simulink model "poles5_rocky"  (R2022a)
settings: Solver=VariableStepAuto  StartTime=0.0  StopTime=5  RelTol=1e-3
values from neighbouring files (symbols this model uses):
  a = 10.12    [poles3_calculate.m]    (also in poles5_calculate.m; poles_calculate.m = 10.33)
  b = 0.00301    [poles3_calculate.m]    (also in poles5_calculate.m; poles_calculate.m = 0.0029)
  Ci_simulink = real(Ci)    [poles5_calculate.m]
  g = 9.81    [poles3_calculate.m]    (also in poles5_calculate.m; poles_calculate.m)
  Ji_simulink = real(Ji)    [poles5_calculate.m]
  Jp_simulink = real(Jp)    [poles5_calculate.m]
  Ki_simulink = real(Ki)    [poles5_calculate.m]
  Kp_simulink = real(Kp)    [poles5_calculate.m]
  l = 0.40038    [poles3_calculate.m]    (also in poles5_calculate.m; poles_calculate.m = 0.4168)
settings Model: Creator=cpark1  LastModifiedBy=cpark1

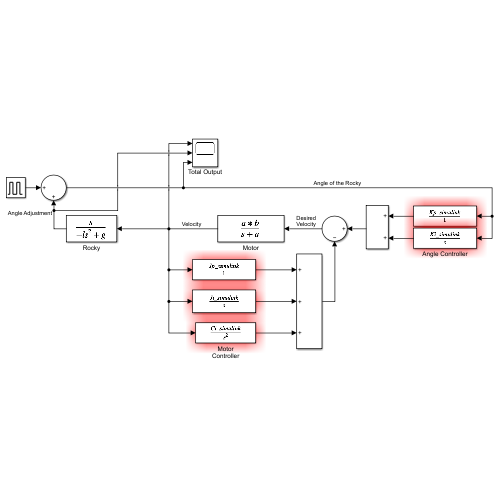
[thumbnail: Simulink's stored preview of the top-level diagram]
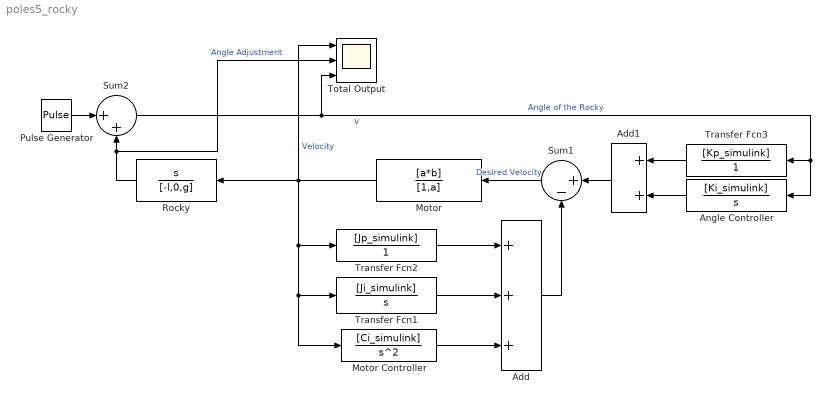
== system poles5_rocky ==
  note: v
  Add : Sum  Inputs=+++
  Add1 : Sum
  Angle Controller : TransferFcn  Numerator=[Ki_simulink]  Denominator=[1 0]
  Motor : TransferFcn  Numerator=[a*b]  Denominator=[1,a]  ContinuousStateAttributes='motor'
  Motor Controller : TransferFcn  Numerator=[Ci_simulink]  Denominator=[1 0 0]
  Pulse Generator : DiscretePulseGenerator  PulseType=Time based  Period=10
  Rocky : TransferFcn  Numerator=[1,0]  Denominator=[-l,0,g]  ContinuousStateAttributes='rocky'
  Sum1 : Sum  Inputs=|+-
  Sum2 : Sum  Inputs=|++
  Total Output : Scope  NumInputPorts=3
  Transfer Fcn1 : TransferFcn  Numerator=[Ji_simulink]  Denominator=[1 0]
  Transfer Fcn2 : TransferFcn  Numerator=[Jp_simulink]  Denominator=[1]
  Transfer Fcn3 : TransferFcn  Numerator=[Kp_simulink]  Denominator=[1]
  wires:
  Pulse Generator/1 -> Sum2/1
  Sum2/1 -> Angle Controller/1, Transfer Fcn3/1, Total Output/3  "Angle of the Rocky"
  Rocky/1 -> Sum2/2, Total Output/2  "Angle Adjustment"
  Sum1/1 -> Motor/1  "Desired Velocity"
  Motor/1 -> Rocky/1, Total Output/1, Transfer Fcn2/1, Transfer Fcn1/1, Motor Controller/1  "Velocity"
  Add/1 -> Sum1/2
  Motor Controller/1 -> Add/3
  Transfer Fcn1/1 -> Add/2
  Transfer Fcn2/1 -> Add/1
  Add1/1 -> Sum1/1
  Transfer Fcn3/1 -> Add1/1
  Angle Controller/1 -> Add1/2
